simulink model "ECE308_4_10"  (R2025a)
settings: Solver=VariableStepAuto  StartTime=0.0  StopTime=10.0  RelTol=1e-3
values from neighbouring files (symbols this model uses):
  d = Z1*conj(Z1)    [ComplexNumbersPolar.m]    (also in ECE308_4.m = 0.03)
  g = -9.8    [ECE308_4.m]    (also in LSPF.m = polyval(P , t1))
  J = 9.99e-6    (= 9.99e-06)    [ECE308_4.m]
  L = 1.0    (= 1)    [ECE308_4.m]    (also in ECE308_ICE.m = (s + 4) / ((s+1)*(s+2)*(s+8)*(s+9)*(s+10)); Lesson23.m = 3; matlab.mat = 3)
  m = p(1)    [ECE302Lab3.m]    (also in ECE308_4.m = 0.111; LSPF.m = 3)
  R = 0.015    [ECE308_4.m]    (also in ECE308_ICE.m = 50; HWMatrix.m = rref(Ab); RREF.m = rref(Ab); SeriesDCMACHINE.m = 7)
settings Model: Creator=cruisemac  LastModifiedBy=cruisemac

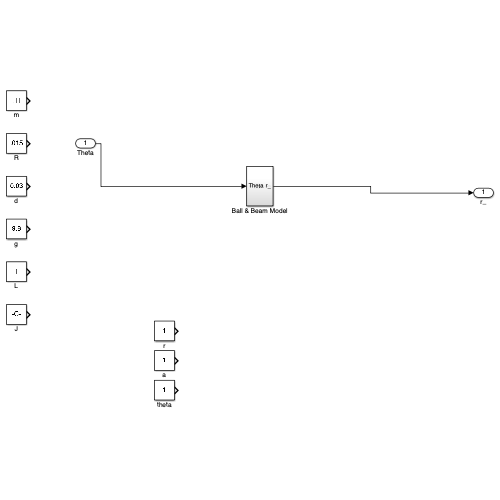
[thumbnail: Simulink's stored preview of the top-level diagram]
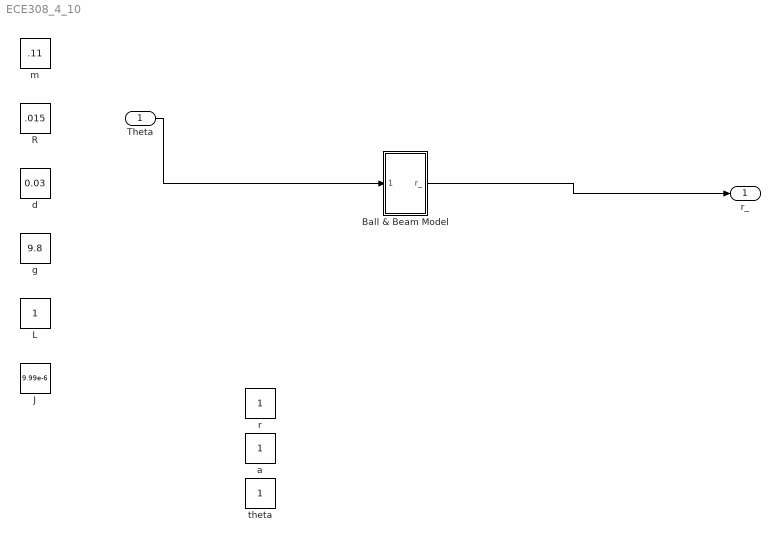
== system ECE308_4_10 ==
  Theta : Inport
  Ball & Beam Model : Subsystem
  J : Constant  Value=9.99e-6
  L : Constant
  R : Constant  Value=.015
  a : Constant
  d : Constant  Value=0.03
  g : Constant  Value=9.8
  m : Constant  Value=.11
  r : Constant
  theta : Constant
  r_ : Outport
  wires:
  Theta/1 -> Ball & Beam Model/1(Theta)
  Ball & Beam Model/1(r_) -> r_/1

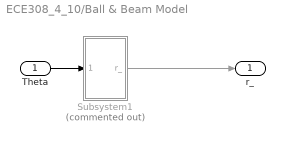
== system ECE308_4_10/Ball & Beam Model ==
  Theta : Inport
  Subsystem1 : Subsystem  Commented=on
  r_ : Outport
  wires:
  Theta/1 -> Subsystem1/1(Theta)
  Subsystem1/1(r_) -> r_/1

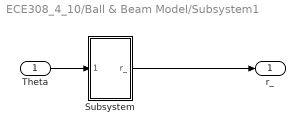
== system ECE308_4_10/Ball & Beam Model/Subsystem1 ==
  Theta : Inport
  Subsystem : Subsystem
  r_ : Outport
  wires:
  Theta/1 -> Subsystem/1(Theta)
  Subsystem/1(r_) -> r_/1

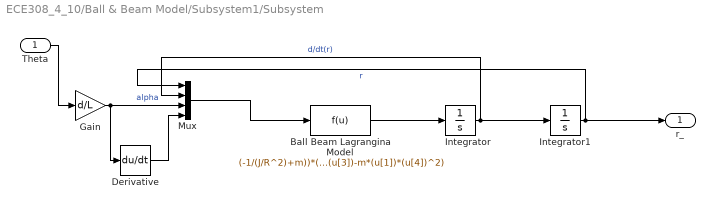
== system ECE308_4_10/Ball & Beam Model/Subsystem1/Subsystem ==
  Theta : Inport
  Ball Beam Lagrangina Model : Fcn  Expr=(-1/(J/R^2)+m))*(m*g*sin(u[3])-m*(u[1])*(u[4])^2)
  Derivative : Derivative
  Gain : Gain  Gain=d/L
  Integrator : Integrator
  Integrator1 : Integrator
  Mux : Mux
  r_ : Outport
  wires:
  Ball Beam Lagrangina Model/1 -> Integrator/1
  Gain/1 -> Derivative/1, Mux/3  "alpha"
  Integrator1/1 -> r_/1, Mux/1  "r"
  Integrator/1 -> Mux/2, Integrator1/1  "d/dt(r)"
  Mux/1 -> Ball Beam Lagrangina Model/1
  Derivative/1 -> Mux/4
  Theta/1 -> Gain/1
